simulink model "SimTrifasicoMeioLinhaComIsolador"  (R2022b)
settings: Solver=ode45  StartTime=0.0  StopTime=SimulacaoTempo  RelTol=1e-3  EnableMultiTasking=on
values from neighbouring files (symbols this model uses):
  C_matrix = [7.14789431755e-09  -2.14393248907e-09; -2.14393248907e-09  7.14789431755e-09]    [Modelo2fios2awg160.mat]    (also in trifasico2awg.mat = [7.86602198725e-09  -2.45195546694e-09  -1.42580481937e-09; ; trifasico2awgNew.mat = [8.93900996847e-09  -2.36457299077e-09  -1.26282974561e-09; )
  dd = [ 20 ]    [CarregaDados20km.m]
  L_matrix = [0.00251001340283  0.00125944754059; 0.00125944754059  0.00251001340283]    [Modelo2fios2awg160.mat]    (also in trifasico2awg.mat = [0.00242085814129  0.00130892171515  0.00117029227904; 0.001; trifasico2awgNew.mat = [0.0018119254645  0.000784575768319  0.000670213848675; 0.00)
  m1 = n    [CurtoCircuitos.m]    (also in CurtosComparadosMonofasicos.m)
  R_matrix = [1.15977689742  0.0576982604784; 0.0576982604784  1.15977689742]    [Modelo2fios2awg160.mat]    (also in trifasico2awg.mat = [1.15895092862  0.0568724513894  0.0568719145431; 0.05687245; trifasico2awgNew.mat = [0.213716566428  0.0989824596492  0.099050906555; 0.09898245)
  Raf = 1e-5    (= 1e-05)    [CurtoCircuitos.m]    (also in CurtosComparadosMonofasicos.m = 1000000)
  Rbf = 1e-5    (= 1e-05)    [CurtoCircuitos.m]    (also in CurtosComparadosMonofasicos.m)
  Rcf = ValorCurto    [CurtoCircuitos.m]    (also in CurtosComparadosMonofasicos.m)
undefined symbols (not defined in the file or in its folder): D11, Delta
libraries: spsSeriesRLCBranchLib x3, spsDistributedParametersLineLib x2, spsThreePhaseVIMeasurementLib x2, spsThreePhaseTransformerTwoWindingsLib x2, spsGroundLib x1, spsThreePhaseSourceLib x1, spspowerguiLib x1
settings Model: Creator=laris  LastModifiedBy=Leonardo Felipe
settings SolverCC: AlgebraicLoopSolver=TrustRegion
settings DataIOCC: LimitDataPoints=on  SaveFormat=Array  ReturnWorkspaceOutputs=off
settings OptimizationCC: LifeSpan=inf
settings DebuggingCC: UnconnectedInputMsg=warning  UnconnectedOutputMsg=warning  UnconnectedLineMsg=warning  SFUnexpectedBacktrackingDiag=warning  SFNoUnconditionalDefaultTransitionDiag=warning  SFExecutionAtInitializationDiag=none  SFMachineParentedDataDiag=warning  ArithmeticOperatorsInVariantConditions=warning
settings HardwareCC: ProdBitPerPointer=32  ProdBitPerSizeT=32  ProdBitPerPtrDiffT=32  ProdLargestAtomicFloat=None  ProdIntDivRoundTo=Undefined  ProdEndianess=Unspecified  ProdWordSize=32  ProdHWDeviceType=32-bit Generic
settings ModelReferenceCC: EnableRefExpFcnMdlSchedulingChecks=on  PropagateSignalLabelsOutOfModel=off
settings SFSimCC: SimUseLocalCustomCode=off  CustomCodeUndefinedFunction=UseInterfaceOnly
settings RTWCC: RTWUseLocalCustomCode=off  DLArmComputeVersion=19.05
settings CodeAppCC: StateflowObjectComments=on
settings GRTTargetCC: TargetLangStandard=C89/C90 (ANSI)
settings ConfigComp: CovMetricSettings=dw  CovSaveCumulativeToWorkspaceVar=on  CovSaveSingleToWorkspaceVar=on  CovExternalEMLEnable=off
settings SimscapeCC: SimscapeNormalizeSystem=off

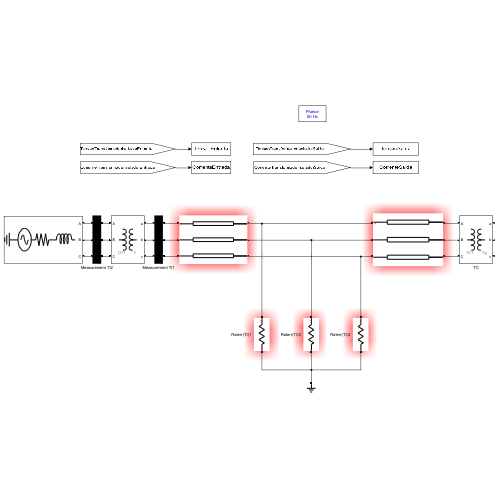
[thumbnail: Simulink's stored preview of the top-level diagram]
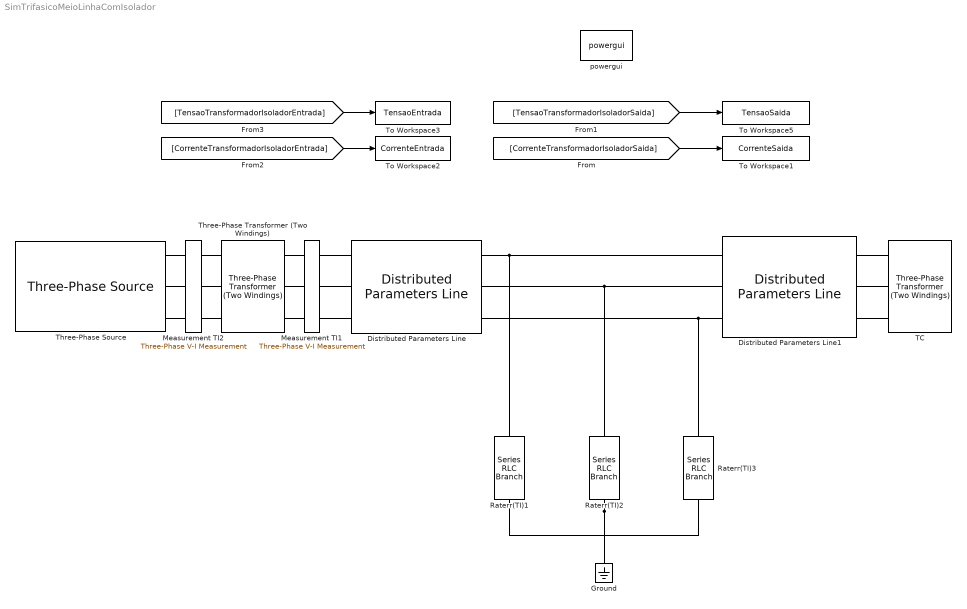
== system SimTrifasicoMeioLinhaComIsolador ==
  Distributed Parameters Line : spsDistributedParametersLineLib/Distributed Parameters Line  Phases=3  Length=dd * m1  Frequency=60  Resistance=R_matrix  Inductance=L_matrix  Capacitance=C_matrix  x1=[374.945996377004 6975.21877840076 4015.31703079136;376.991118430775 376.991118430775 376.991118430775;-1.57668915249281 -1.57281888382336 -1.57296826950161]  x2=[374.971653263932 6974.74174001446 4016.16117651489;376.991118430775 376.991118430775 376.991118430775;-1.57654474518852 -1.5728638973592 -1.57285286189856]  x3=[4.76600739733514 60.7842187606867 149.610840727795;376.991118430775 376.991118430775 376.991118430775;-1.43109782967936 1.80198089003186 -1.43342770822003]  x4=[4.11383733247366 98.1734043528426 124.096021303055;376.991118430775 376.991118430775 376.991118430775;1.73377091492178 -1.42925108719572 1.73709441776477]  x5=2.60355177502627e-08  V1=ones(3,3)  V2=ones(3,3)  I1=ones(3,3)  I2=ones(3,3)  nHarmo=1  Measurements=None  Decoupling=on  VsMag0=[3432.94160851137 3431.5677302442 6431.50745940818]  VrMag0=[3432.25924099268 3432.25703133477 6431.51526410914]  VsAngle0=[-90.124850469061 -90.1380748033708 89.8895796476869]  VrAngle0=[-90.1313448722152 -90.1313508240354 89.8890890163282]  IsMag0=[104.020722805163 122.149404473617 18.7960868730939]  IrMag0=[120.042134396798 101.414500177135 18.8461221506428]  IsAngle0=[100.085986055351 -82.1257785221161 85.4820228207952]  IrAngle0=[-81.2878057930745 99.5239794669207 94.2743222537898]
  Distributed Parameters Line1 : spsDistributedParametersLineLib/Distributed Parameters Line  Phases=3  Length=dd * (1-m1)  Frequency=60  Resistance=R_matrix  Inductance=L_matrix  Capacitance=C_matrix  x1=[374.971653263932 6974.74174001446 4016.16117651489;376.991118430775 376.991118430775 376.991118430775;-1.67467670442656 -1.64995412698105 -1.65029763278064]  x2=[376.761364257887 6994.7440826184 4027.77187710346;376.991118430775 376.991118430775 376.991118430775;-1.67799576797381 -1.65689613407413 -1.65852034245761]  x3=[0.31535986234065 16.6633665135179 11.0491076885258;376.991118430775 376.991118430775 376.991118430775;-1.77421387408245 -1.73028278987777 -1.73166207766748]  x4=[0.315650431884567 16.6781551901588 11.0578447135983;376.991118430775 376.991118430775 376.991118430775;-1.6782969558481 -1.657183273791 -1.65876628432774]  x5=0.000260329141984877  V1=ones(3,3)  V2=ones(3,3)  I1=ones(3,3)  I2=ones(3,3)  nHarmo=1  Measurements=None  Decoupling=on  VsMag0=[3432.25924099268 3432.25703133477 6431.51526410914]  VrMag0=[3442.4696370778 3442.60759757331 6449.59335627727]  VsAngle0=[-90.1313448722152 -90.1313508240354 89.8890890163282]  VrAngle0=[-90.4796968846104 -90.5839118041366 89.4649775259642]  IsMag0=[7.83490106765077 9.99392068590532 17.9544179530586]  IrMag0=[7.84241995133601 10.001894811566 17.9697906603488]  IsAngle0=[-94.7119638394192 -94.8038081522872 85.2757539811987]  IrAngle0=[-90.4852191001945 -90.6013019992422 89.4472664815979]
  Ground : spsGroundLib/Ground  LConnTagsString=a
  Measurement TI1 : spsThreePhaseVIMeasurementLib/Three-Phase V-I Measurement  VoltageMeasurement=phase-to-phase  SetLabelV=on  LabelV=TensaoTransformadorIsoladorSaida  Vpu=off  VpuLL=off  CurrentMeasurement=yes  SetLabelI=on  LabelI=CorrenteTransformadorIsoladorSaida  Ipu=off  Pbase=100e6  Vbase=500e3  OutputType=Complex  PhasorSimulation=on  PSBequivalent=0
  Measurement TI2 : spsThreePhaseVIMeasurementLib/Three-Phase V-I Measurement  VoltageMeasurement=phase-to-phase  SetLabelV=on  LabelV=TensaoTransformadorIsoladorEntrada  Vpu=off  VpuLL=off  CurrentMeasurement=yes  SetLabelI=on  LabelI=CorrenteTransformadorIsoladorEntrada  Ipu=off  Pbase=100e6  Vbase=500e3  OutputType=Complex  PhasorSimulation=on  PSBequivalent=0
  Raterr(TI)1 : spsSeriesRLCBranchLib/Series RLC Branch  LConnTagsString=__new0  RConnTagsString=__new0  BranchType=R  Resistance=Raf  Inductance=0  SetiL0=off  InitialCurrent=0  Capacitance=1e-6  Setx0=off  InitialVoltage=0  Measurements=None
  Raterr(TI)2 : spsSeriesRLCBranchLib/Series RLC Branch  LConnTagsString=__new0  RConnTagsString=__new0  BranchType=R  Resistance=Rbf  Inductance=0  SetiL0=off  InitialCurrent=0  Capacitance=1e-6  Setx0=off  InitialVoltage=0  Measurements=None
  Raterr(TI)3 : spsSeriesRLCBranchLib/Series RLC Branch  LConnTagsString=__new0  RConnTagsString=__new0  BranchType=R  Resistance=Rcf  Inductance=0  SetiL0=off  InitialCurrent=0  Capacitance=1e-6  Setx0=off  InitialVoltage=0  Measurements=None
  TC : spsThreePhaseTransformerTwoWindingsLib/Three-Phase Transformer (Two Windings)  Winding1Connection=Delta (D11)  Winding2Connection=Yg  CoreType=Three single-phase transformers  SetSaturation=off  Hysteresis=off  DataFile='hysteresis'  SetInitialFlux=off  Measurements=None  UNITS=pu  NominalPower=[120e3 , 60]  Winding1=[13800 0.0048118 0.018511]  Winding2=[380 0.0048119 0.018511]  Rm=5.801193266567229e+02  Lm=8.409977380031759e+02  L0=0.50001  Saturation=[0 0;0.0012545 0.01913;0.52272 0.024231]  InitialFluxes=[0.66025 -0.66025 0.57768]  BreakLoop=off  DiscreteSolver=Trapezoidal iterative  DataType=off  TransfoNumber=1
  Three-Phase Transformer (Two Windings) : spsThreePhaseTransformerTwoWindingsLib/Three-Phase Transformer (Two Windings)  Winding1Connection=Delta (D11)  Winding2Connection=Y  CoreType=Three single-phase transformers  SetSaturation=off  Hysteresis=off  DataFile='hysteresis'  SetInitialFlux=off  Measurements=None  UNITS=pu  NominalPower=[120e3 , 60 ]  Winding1=[13800 0.004 0.023]  Winding2=[13800/sqrt(3) 0.004 0.023]  Rm=500  Lm=500  L0=0.5  Saturation=[0 0;0.0024 1.2;1 1.52]  InitialFluxes=[ 0.8 , -0.8 , 0.7 ]  BreakLoop=off  DiscreteSolver=Trapezoidal iterative  DataType=off  TransfoNumber=1
  Three-Phase Source : spsThreePhaseSourceLib/Three-Phase Source  InternalConnection=Yg  VoltagePhases=off  Voltage=13.8e3  PhaseAngle=0  Voltage_phases=[25e3 25e3 25e3]/sqrt(3)  PhaseAngles_phases=[0 -120 +120]  Frequency=60  NonIdealSource=on  SpecifyImpedance=on  Resistance=0.8929  Inductance=16.58e-3  ShortCircuitLevel=7.2e6  BaseVoltage=13.8e3  XRratio=7  BusType=swing  Pref=10e3  Qref=0  Prefabc=[10e3, 10e3, 10e3]  Qrefabc=[0, 0, 0]  Qmin=-inf  Qmax=inf
  To Workspace1 : ToWorkspace  VariableName=CorrenteSaida  SampleTime=-1
      settings: MaxDataPoints=1
  To Workspace2 : ToWorkspace  VariableName=CorrenteEntrada  SampleTime=-1
      settings: MaxDataPoints=1
  To Workspace3 : ToWorkspace  VariableName=TensaoEntrada  SampleTime=-1
      settings: MaxDataPoints=1
  To Workspace5 : ToWorkspace  VariableName=TensaoSaida  SampleTime=-1
      settings: MaxDataPoints=1
  powergui : spspowerguiLib/powergui  Priority=1  SimulationMode=Phasor  SampleTime=50e-9  frequency=60  Iterations=50  frequencyindice=60  Pbase=100e6  ErrMax=1e-4  UnitsV=kV  UnitsW=MW  buscounter=0  FunctionMessages=off  echomessages=off  EnableUseOfTLC=off  CurrentSourceSwitches=off  DisableSnubberDevices=off  DisableRonSwitches=off  DisableVfSwitches=off  DisplayEquations=off  AutomaticDiscreteSolvers=off  SolverType=Tustin/Backward Euler (TBE)  Interpol=off  ExternalGateDelay=off  methode=off  Ts=100  x0status=blocks  SPID=on  SwTol=0  HookPort=off  NonlinearTolerance=1e-4  nMaxIteration=100  ContinueOnMaxIteration=off  RestoreLinks=warning  ResistiveCurrentMeasurement=off  Frange=[0:2:500]  Ylog=off  Xlog=on  ShowGrid=off  save=off  variable=ZData  structure=0  ZoomFFT=off  StartTime=0.0  cycles=1  DisplayStyle=1  fundamental=60  FreqAxis=off  MaxFrequency=1000  frequencyindicesteady=1  RmsSteady=1  display=off
  wires:
  [CorrenteTransformadorIsoladorSaida] -> To Workspace1/1
  [TensaoTransformadorIsoladorSaida] -> To Workspace5/1
  [CorrenteTransformadorIsoladorEntrada] -> To Workspace2/1
  [TensaoTransformadorIsoladorEntrada] -> To Workspace3/1
  connections:
  Distributed Parameters Line1/LConn2 -- Raterr(TI)2/LConn1 -- Distributed Parameters Line/RConn2
  Distributed Parameters Line1/RConn1 -- TC/LConn1
  Distributed Parameters Line1/RConn2 -- TC/LConn2
  Distributed Parameters Line1/RConn3 -- TC/LConn3
  Distributed Parameters Line/LConn3 -- Measurement TI1/RConn3
  Distributed Parameters Line1/LConn3 -- Raterr(TI)3/LConn1 -- Distributed Parameters Line/RConn3
  Distributed Parameters Line/LConn1 -- Measurement TI1/RConn1
  Distributed Parameters Line/LConn2 -- Measurement TI1/RConn2
  Distributed Parameters Line1/LConn1 -- Raterr(TI)1/LConn1 -- Distributed Parameters Line/RConn1
  Raterr(TI)2/RConn1 -- Ground/LConn1 -- Raterr(TI)1/RConn1 -- Raterr(TI)3/RConn1
  Three-Phase Transformer (Two Windings)/RConn1 -- Measurement TI1/LConn1
  Measurement TI1/LConn2 -- Three-Phase Transformer (Two Windings)/RConn2
  Three-Phase Transformer (Two Windings)/RConn3 -- Measurement TI1/LConn3
  Measurement TI2/RConn1 -- Three-Phase Transformer (Two Windings)/LConn1
  Measurement TI2/RConn2 -- Three-Phase Transformer (Two Windings)/LConn2
  Measurement TI2/RConn3 -- Three-Phase Transformer (Two Windings)/LConn3
  Three-Phase Source/RConn2 -- Measurement TI2/LConn2
  Three-Phase Source/RConn1 -- Measurement TI2/LConn1
  Three-Phase Source/RConn3 -- Measurement TI2/LConn3
